simulink model "project2_week_1"  (R2020b)
settings: Solver=VariableStepAuto  StartTime=0.0  StopTime=10.0  RelTol=1e-3
undefined symbols (not defined in the file): b, k1, K2
settings Model: Creator=RASIKA MALGI  LastModifiedBy=RASIKA MALGI

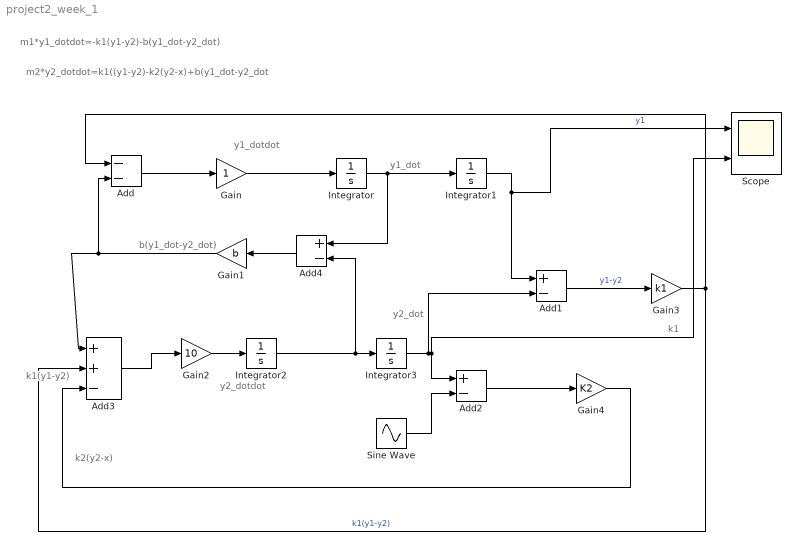
== system project2_week_1 ==
  note: m2*y2_dotdot=k1((y1-y2)-k2(y2-x)+b(y1_dot-y2_dot
  note: m1*y1_dotdot=-k1(y1-y2)-b(y1_dot-y2_dot)
  note: b(y1_dot-y2_dot)
  note: k1(y1-y2)
  note: k2(y2-x)
  note: y2_dotdot
  note: y2_dot
  note: k1
  note: y1_dot
  note: y1_dotdot
  Add : Sum  Inputs=--
  Add1 : Sum  Inputs=+-
  Add2 : Sum  Inputs=+-
  Add3 : Sum  Inputs=++-
  Add4 : Sum  Inputs=+-
  Gain : Gain
  Gain1 : Gain  Gain=b
  Gain2 : Gain  Gain=10
  Gain3 : Gain  Gain=k1
  Gain4 : Gain  Gain=K2
  Integrator{,1..3} (4 alike) : Integrator
  Scope : Scope  NumInputPorts=2
  Sine Wave : Sin  SampleTime=0
  wires:
  Add3/1 -> Gain2/1
  Gain2/1 -> Integrator2/1
  Integrator2/1 -> Add4/2, Integrator3/1
  Add/1 -> Gain/1
  Gain/1 -> Integrator/1
  Integrator/1 -> Add4/1, Integrator1/1
  Add1/1 -> Gain3/1  "y1-y2"
  Add4/1 -> Gain1/1
  Integrator3/1 -> Add1/2, Add2/1, Scope/2
  Add2/1 -> Gain4/1
  Gain1/1 -> Add/2, Add3/1
  Gain4/1 -> Add3/3
  Sine Wave/1 -> Add2/2
  Gain3/1 -> Add3/2, Add/1  "k1(y1-y2)"
  Integrator1/1 -> Scope/1, Add1/1  "y1"
